simulink library "ArdupilotFunctions"  (R2024a)
settings: Solver=VariableStepAuto  StartTime=0.0  StopTime=10.0  RelTol=1e-3
undefined symbols (not defined in the file): AltHold_Freq, DiscIntNeverNeededParam, PSC_VELZ_D, PSC_VELZ_FF, PSC_VELZ_FLTD, PSC_VELZ_FLTE, PSC_VELZ_I, PSC_VELZ_IMAX, PSC_VELZ_P
libraries: eeGeneralControl x5, simulink x3
settings Model: Creator=igmso  LastModifiedBy=igmso

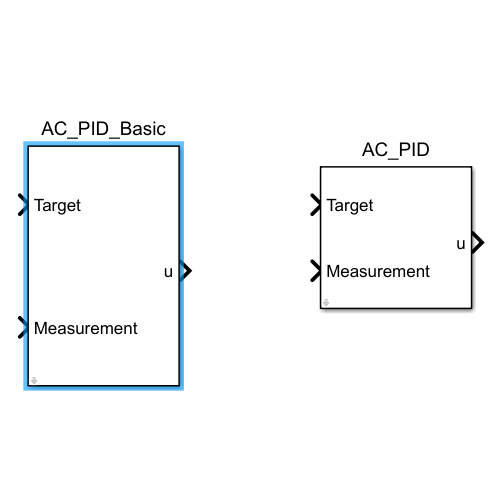
[thumbnail: Simulink's stored preview of the top-level diagram]
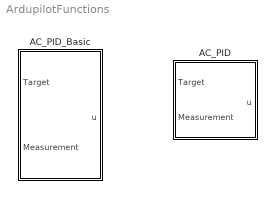
== system ArdupilotFunctions ==
  AC_PID : Subsystem  mask{P=1, I=1, D=1, FF=1, D_FF=1, FLTD=1, FLTE=1, FLTT=1, IMAX=1}
      mask prompts: P "Proportional Gain:"; I "Integral Gain:"; D "Derivative Gain:"; FF "FeedForward Gain:"; D_FF "Derivative FeedForward Gain:"; FLTD "Controller Derivative Frequency in Hz:"; FLTE "Controller Error Frequency in Hz:"; FLTT "Controller Target Frequency in Hz:"; IMAX "Integral Gain Maximum:"
  AC_PID_Basic : Subsystem  mask{P=PSC_VELZ_P, I=PSC_VELZ_I, D=PSC_VELZ_D, FF=PSC_VELZ_FF, FLTD=PSC_VELZ_FLTD, FLTE=PSC_VELZ_FLTE, IMAX=PSC_VELZ_IMAX}
      mask prompts: P "Proportional Gain:"; I "Integral Gain:"; D "Derivative Gain:"; FF "FeedForward Gain :"; FLTD "Controller Derivative Frequency in Hz:"; FLTE "Controller Error Frequency in Hz:"; IMAX "Integral Gain Maximum:"

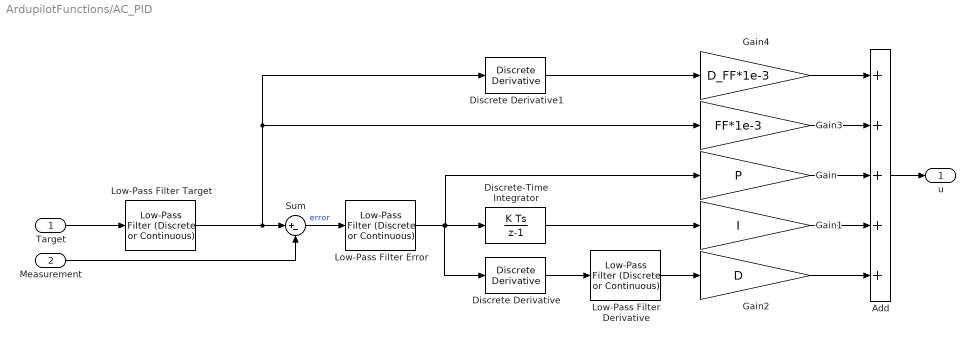
== system ArdupilotFunctions/AC_PID ==
  Target : Inport
  Measurement : Inport  Port=2
  Add : Sum  Inputs=5
  Discrete Derivative : simulink/Discrete/Discrete Derivative  gainval=1.0  ICPrevScaledInput=0.0  OutMin=[]  OutMax=[]  OutDataType=fixdt(1, 16)  OutScaling=2^-10  DoSatur=off
  Discrete Derivative1 : simulink/Discrete/Discrete Derivative  gainval=1.0  ICPrevScaledInput=0.0  OutMin=[]  OutMax=[]  OutDataType=fixdt(1, 16)  OutScaling=2^-10  DoSatur=off
  Discrete-Time Integrator : DiscreteIntegrator  SampleTime=1/AltHold_Freq  LimitOutput=on  UpperSaturationLimit=IMAX  LowerSaturationLimit=-IMAX  StateName='Accel_Z_I'  ICPrevOutput=DiscIntNeverNeededParam  ICPrevScaledInput=DiscIntNeverNeededParam
  Gain : Gain  Gain=P
  Gain1 : Gain  Gain=I
  Gain2 : Gain  Gain=D
  Gain3 : Gain  Gain=FF*1e-3
  Gain4 : Gain  Gain=D_FF*1e-3
  Low-Pass Filter Derivative : eeGeneralControl/Low-Pass Filter (Discrete or Continuous)  K=1  T=1/(2*pi*FLTD)  B=inf  A=-inf  init_option=Inherited from block input  x0=0  Ts=1/AltHold_Freq
  Low-Pass Filter Error : eeGeneralControl/Low-Pass Filter (Discrete or Continuous)  K=1  T=1/(2*pi*FLTE)  B=inf  A=-inf  init_option=Inherited from block input  x0=0  Ts=1/AltHold_Freq
  Low-Pass Filter Target : eeGeneralControl/Low-Pass Filter (Discrete or Continuous)  K=1  T=1/(2*pi*FLTT)  B=inf  A=-inf  init_option=Inherited from block input  x0=0  Ts=1/AltHold_Freq
  Sum : Sum  Inputs=|+-
  u : Outport
  wires:
  Gain4/1 -> Add/1
  Discrete Derivative1/1 -> Gain4/1
  Low-Pass Filter Target/1 -> Sum/1, Discrete Derivative1/1, Gain3/1
  Add/1 -> u/1
  Gain2/1 -> Add/5
  Gain3/1 -> Add/2
  Gain1/1 -> Add/4
  Gain/1 -> Add/3
  Low-Pass Filter Derivative/1 -> Gain2/1
  Discrete-Time Integrator/1 -> Gain1/1
  Discrete Derivative/1 -> Low-Pass Filter Derivative/1
  Low-Pass Filter Error/1 -> Discrete Derivative/1, Gain/1, Discrete-Time Integrator/1
  Sum/1 -> Low-Pass Filter Error/1  "error"
  Measurement/1 -> Sum/2
  Target/1 -> Low-Pass Filter Target/1

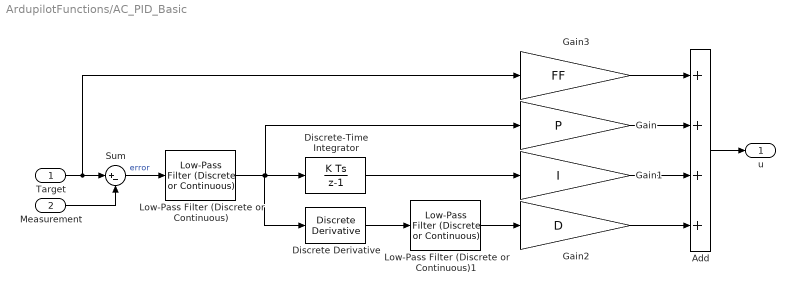
== system ArdupilotFunctions/AC_PID_Basic ==
  Target : Inport
  Measurement : Inport  Port=2
  Add : Sum  Inputs=4
  Discrete Derivative : simulink/Discrete/Discrete Derivative  gainval=1.0  ICPrevScaledInput=0.0  OutMin=[]  OutMax=[]  OutDataType=fixdt(1, 16)  OutScaling=2^-10  DoSatur=off
  Discrete-Time Integrator : DiscreteIntegrator  SampleTime=1/AltHold_Freq  LimitOutput=on  UpperSaturationLimit=IMAX  LowerSaturationLimit=-IMAX  StateName='Vel_z_I'  ICPrevOutput=DiscIntNeverNeededParam  ICPrevScaledInput=DiscIntNeverNeededParam
  Gain : Gain  Gain=P
  Gain1 : Gain  Gain=I
  Gain2 : Gain  Gain=D
  Gain3 : Gain  Gain=FF
  Low-Pass Filter (Discrete or Continuous) : eeGeneralControl/Low-Pass Filter (Discrete or Continuous)  K=1  T=1/(2*pi*FLTE)  B=inf  A=-inf  init_option=Inherited from block input  x0=0  Ts=1/AltHold_Freq
  Low-Pass Filter (Discrete or Continuous)1 : eeGeneralControl/Low-Pass Filter (Discrete or Continuous)  K=1  T=1/(2*pi*FLTD)  B=inf  A=-inf  init_option=Inherited from block input  x0=0  Ts=1/AltHold_Freq
  Sum : Sum  Inputs=|+-
  u : Outport
  wires:
  Target/1 -> Gain3/1, Sum/1
  Measurement/1 -> Sum/2
  Sum/1 -> Low-Pass Filter (Discrete or Continuous)/1  "error"
  Low-Pass Filter (Discrete or Continuous)/1 -> Discrete-Time Integrator/1, Gain/1, Discrete Derivative/1
  Discrete Derivative/1 -> Low-Pass Filter (Discrete or Continuous)1/1
  Discrete-Time Integrator/1 -> Gain1/1
  Low-Pass Filter (Discrete or Continuous)1/1 -> Gain2/1
  Gain/1 -> Add/2
  Gain1/1 -> Add/3
  Gain3/1 -> Add/1
  Gain2/1 -> Add/4
  Add/1 -> u/1
